simulink model "TestcmplxPL_example"  (R2017a)
settings: Solver=ode3  StartTime=0.0  StopTime=1000  FixedStep=1  RelTol=1e-3  EnableMultiTasking=on
libraries: Lib_PF_ImpedanceAC_TMATS x3, Lib_PF_BusGenAC_TMATS x1, Lib_PF_BusLoadAC_TMATS x1, Lib_Solve_SSNRSolverJC_TMATS x1, Lib_PF_BusSlackAC_TMATS x1
settings Model: Creator=jwchapm2  LastModifiedBy=glthoma1
settings DataIOCC: LimitDataPoints=on  SaveFormat=Array
settings OptimizationCC: LifeSpan=inf
settings DebuggingCC: SFUnexpectedBacktrackingDiag=warning  SFNoUnconditionalDefaultTransitionDiag=warning  SFExecutionAtInitializationDiag=none
settings HardwareCC: ProdBitPerPointer=32  ProdBitPerSizeT=32  ProdBitPerPtrDiffT=32  ProdLargestAtomicFloat=None  ProdIntDivRoundTo=Undefined  ProdEndianess=Unspecified  ProdWordSize=32  ProdHWDeviceType=32-bit Generic
settings ModelReferenceCC: PropagateSignalLabelsOutOfModel=off
settings GRTTargetCC: TargetLangStandard=C89/C90 (ANSI)  GeneratePreprocessorConditionals=Disable all
settings ConfigComp: CovMetricSettings=dw  CovHtmlReporting=on  CovSaveCumulativeToWorkspaceVar=on  CovSaveSingleToWorkspaceVar=on  CovExternalEMLEnable=off

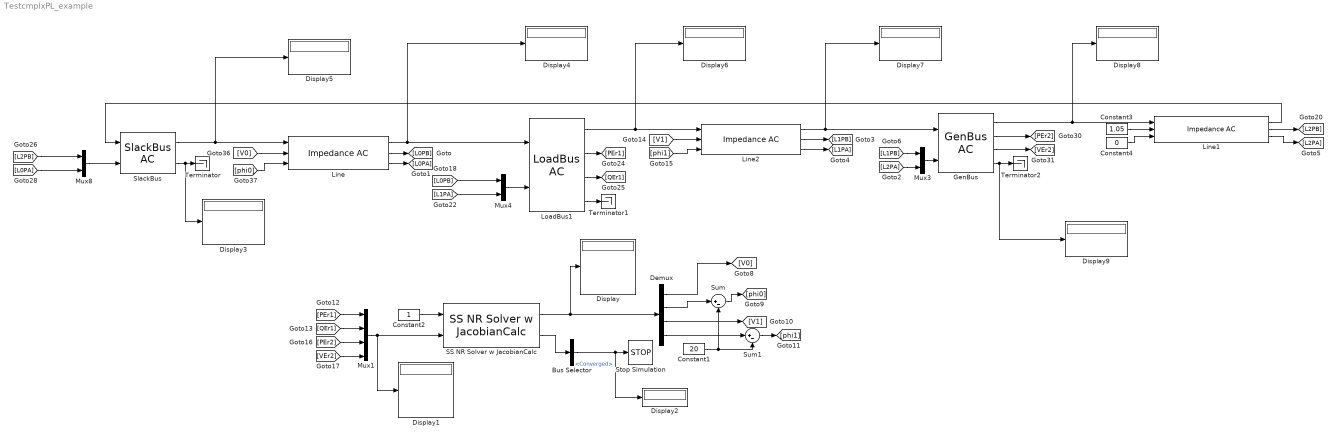
== system TestcmplxPL_example ==
  Bus Selector : BusSelector  OutputSignals=Converged
  Constant1 : Constant  Value=20
  Constant2 : Constant
  Constant3 : Constant  Value=1.05
  Constant4 : Constant  Value=0
  Demux : Demux
  Display{,1..9} (10 alike) : Display
  GenBus : Lib_PF_BusGenAC_TMATS/GenBus AC  PeInEN_M=off  BlkNm_M=double(gcb)  Vispec_M=1.04  P_M=2  Qmax_M=100  Qmin_M=-100
  Line : Lib_PF_ImpedanceAC_TMATS/Impedance AC  R_M=0.02  X_M=0.04
  Line1 : Lib_PF_ImpedanceAC_TMATS/Impedance AC  R_M=0.01  X_M=0.03
  Line2 : Lib_PF_ImpedanceAC_TMATS/Impedance AC  R_M=0.0125  X_M=0.025
  LoadBus1 : Lib_PF_BusLoadAC_TMATS/LoadBus AC  PeInEN_M=off  P_M=-4  QeInEN_M=off  Q_M=-2.5  BlkNm_M=double(gcb)
  Mux1 : Mux
  Mux3 : Mux  Inputs=2
  Mux4 : Mux  Inputs=2
  Mux8 : Mux  Inputs=2
  SS NR Solver w JacobianCalc : Lib_Solve_SSNRSolverJC_TMATS/SS NR Solver w JacobianCalc  SJac_Per_M=[0.01 0.01 0.01 0.01;-0.01 -0.01,-0.01,-0.01]  SNR_IC_M=[1,20 , 1.04, 20]  SNR_DX_M=5  SNR_Mx_M=100000  SNR_Mn_M=0.00001  SJacobianAttempts_M=20  Cond_Limits_M=0.000001
  SlackBus : Lib_PF_BusSlackAC_TMATS/SlackBus AC
  Stop Simulation : Stop
  Sum : Sum  Inputs=|+-
  Sum1 : Sum  Inputs=|+-
  Terminator : Terminator
  Terminator1 : Terminator
  Terminator2 : Terminator
  wires:
  SlackBus/1 -> Display5/1, Line/1
  Line/1 -> LoadBus1/1, Display4/1
  SlackBus/2 -> Display3/1, Terminator/1
  Line/2 -> [L0PB]
  Line1/2 -> [L2PB]
  [L2PB] -> Mux8/1
  [L0PA] -> Mux8/2
  Mux8/1 -> SlackBus/2
  [V0] -> Line/2
  [phi0] -> Line/3
  Constant3/1 -> Line1/2
  Constant4/1 -> Line1/3
  SS NR Solver w JacobianCalc/2 -> Bus Selector/1
  Bus Selector/1 -> Display2/1, Stop Simulation/1  "<Converged>"
  Demux/2 -> Sum/1
  Demux/1 -> [V0]
  Demux/4 -> Sum1/1
  Demux/3 -> [V1]
  [PEr1] -> Mux1/1
  [QEr1] -> Mux1/2
  [PEr2] -> Mux1/3
  [VEr2] -> Mux1/4
  Mux1/1 -> Display1/1, SS NR Solver w JacobianCalc/2
  Constant2/1 -> SS NR Solver w JacobianCalc/1
  SS NR Solver w JacobianCalc/1 -> Demux/1, Display/1
  Mux4/1 -> LoadBus1/2
  Line2/3 -> [L1PA]
  [V1] -> Line2/2
  [phi1] -> Line2/3
  LoadBus1/1 -> Display6/1, Line2/1
  [L0PB] -> Mux4/1
  [L1PA] -> Mux4/2
  GenBus/1 -> Line1/1, Display8/1
  Line2/1 -> GenBus/1, Display7/1
  Mux3/1 -> GenBus/2
  [L1PB] -> Mux3/1
  [L2PA] -> Mux3/2
  LoadBus1/2 -> [PEr1]
  LoadBus1/3 -> [QEr1]
  LoadBus1/4 -> Terminator1/1
  GenBus/2 -> [PEr2]
  GenBus/3 -> [VEr2]
  GenBus/4 -> Display9/1, Terminator2/1
  Line1/1 -> SlackBus/1
  Sum/1 -> [phi0]
  Sum1/1 -> [phi1]
  Constant1/1 -> Sum1/2, Sum/2
  Line/3 -> [L0PA]
  Line2/2 -> [L1PB]
  Line1/3 -> [L2PA]
